simulink model "lorenz_model"  (R2024b)
settings: Solver=ode1  StartTime=0.0  StopTime=40  FixedStep=0.001  MaxStep=0.01  RelTol=1e-3
undefined symbols (not defined in the file or in its folder): beta, rho, sigma

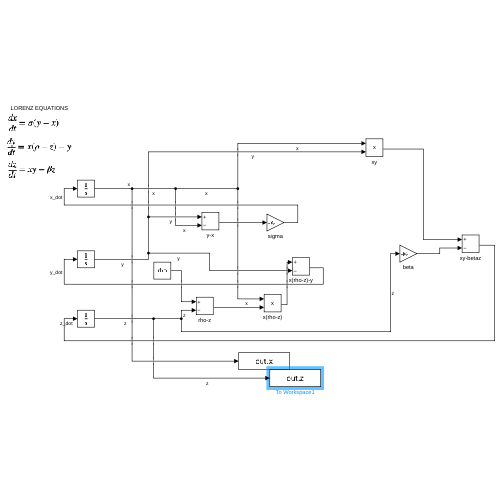
[thumbnail: Simulink's stored preview of the top-level diagram]
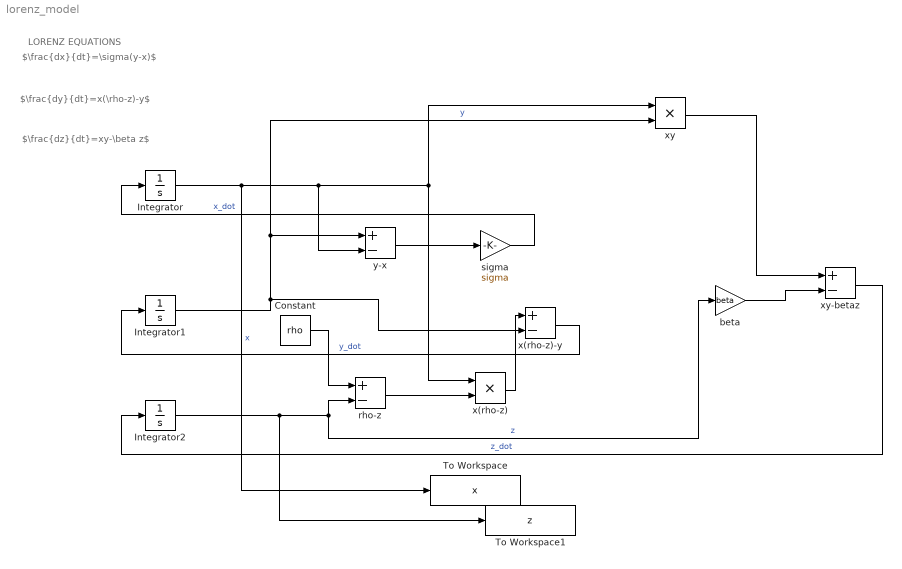
== system lorenz_model ==
  note: LORENZ EQUATIONS
  note: $\frac{dz}{dt}=xy-\beta z$
  note: $\frac{dy}{dt}=x(\rho-z)-y$
  note: $\frac{dx}{dt}=\sigma(y-x)$
  Constant : Constant  Value=rho
  Integrator : Integrator  InitialCondition=1
  Integrator1 : Integrator  InitialCondition=1
  Integrator2 : Integrator  InitialCondition=1
  To Workspace : ToWorkspace  VariableName=x  SampleTime=-1
  To Workspace1 : ToWorkspace  VariableName=z  SampleTime=-1
  beta : Gain  Gain=beta
  rho-z : Sum  Inputs=+-
  sigma : Gain  Gain=sigma
  x(rho-z) : Product
  x(rho-z)-y : Sum  Inputs=+-
  xy : Product
  xy-betaz : Sum  Inputs=+-
  y-x : Sum  Inputs=+-
  wires:
  sigma/1 -> Integrator/1  "x_dot"
  Integrator/1 -> To Workspace/1, xy/1, x(rho-z)/1, y-x/2  "x"
  x(rho-z)-y/1 -> Integrator1/1  "y_dot"
  Integrator1/1 -> x(rho-z)-y/2, xy/2, y-x/1  "y"
  xy-betaz/1 -> Integrator2/1  "z_dot"
  Integrator2/1 -> To Workspace1/1, beta/1, rho-z/2  "z"
  y-x/1 -> sigma/1
  Constant/1 -> rho-z/1
  rho-z/1 -> x(rho-z)/2
  x(rho-z)/1 -> x(rho-z)-y/1
  xy/1 -> xy-betaz/1
  beta/1 -> xy-betaz/2
